simulink model "Ensamblaje_pendulo_furuta_multibody_v4"  (R2025a)
settings: Solver=ode4  StartTime=0.0  StopTime=60  FixedStep=0.002  RelTol=1e-3
PreLoadFcn:
  | d=fileparts(get_param('Ensamblaje_pendulo_furuta_multibody_v4','FileName')); while ~isempty(d)&&~isfile(fullfile(d,'setup_paths.m')), n=fileparts(d); if strcmp(n,d),break;end; d=n; end; if isfile(fullfile(d,'setup_paths.m')), addpath(d); setup_paths; end
  | setup_swingup_quanser; Ensamblaje_pendulo_furuta_multibody_v4_DataFile;
InitFcn:
  | setup_swingup_quanser; Ensamblaje_pendulo_furuta_multibody_v4_DataFile;
model workspace: external: MATLAB File C:\Users\sebas\Documents\TESIS\Scape\Ensamblaje_pendulo_furuta_multibody_v4_DataFile.m (data not in the file)
undefined symbols (not defined in the file): g, Jp_cm, kt, l, mp, mr, r, Rm
libraries: fl_lib x6, simulink_extras x6, nesl_utility x6, simulink x5, sm_lib x2, ee_lib x1
settings Model: Creator=sebas  LastModifiedBy=sebas
settings ExplorerConfigSet: InternalSimMechanicsExplorerSettings=|
  | <ExplorerConfiguration>
  | 
  |   <canonicalview>planar_xy</canonicalview>
  | 
  |   <TilePanel>
  |     <TileInfo>
  |       <Tiles Columns="1" Count="1" Height="592" Rows="1" Width="1064">
  |         <Row Weight="1"/>
  |         <Column Weight="1"/>
  |         <Tile Height="1" Width="1" X="0" Y="0"/>
  |       </Tiles>
  |     </TileInfo>
  |     <SceneInfo>
  |       <SceneViewer>
  |         <IsThisViewStd>
  |           <IsStandardView>off</IsStandardView>
  |           <StandardViewName>Front</StandardViewName>
  |         </IsThisViewStd>
  |         <BGColor>
  |           <R>1</R>
  |           <G>1</G>
  |           <B>1</B>
  |           <A>1</A>
  |         </BGColor>
  |         <Camera>
  |           <DoPerspective>off</DoPerspective>
  |           <Position>
  |             <X>0.15562955258539984</X>
  |             <Y>0.44865320150635074</Y>
  |             <Z>-0.59717677203901176</Z>
  |           </Position>
  |           <Center>
  |             <X>-0.047110070178558651</X>
  |             <Y>0.055245833996093285</Y>
  |             <Z>0.019492845057677309</Z>
  |           </Center>
  |           <Up>
  |             <X>-0.56022370531309607</X>
  |             <Y>0.7694686491141598</Y>
  |             <Z>0.30670408871695148</Z>
  |           </Up>
  |           <XLim>0.11928668495035986</XLim>
  |           <YLim>0.11928668495035986</YLim>
  |           <ViewLimDist>0.01</ViewLimDist>
  |         </Camera>
  |       </SceneViewer>
  |     </SceneInfo>
  |   </TilePanel>
  | 
  |   <MechEditorPanel>
  |     <GfxPanelCameraMap/>
  |     <Cameras/>
  |     <VideoCreator>
  |       <IncludeTiles>All</IncludeTiles>
  |       <IncludeTime>on</IncludeTime>
  |       <IncludeWorldFrame>off</IncludeWorldFrame>
  |       <PlaybackSpeedRatio>1</PlaybackSpeedRatio>
  |       <FrameRate>30</FrameRate>
  |       <FrameSize>auto</FrameSize>
  |       <VideoFormat>UncompressedAVI</VideoFormat>
  |     </VideoCreator>
  |   </MechEditorPanel>
  | 
  |   <PlaybackSettings>
  |     <PlaybackSpeedFactor>1</PlaybackSpeedFactor>
  |   </PlaybackSettings>
  | 
  | </ExplorerConfiguration>

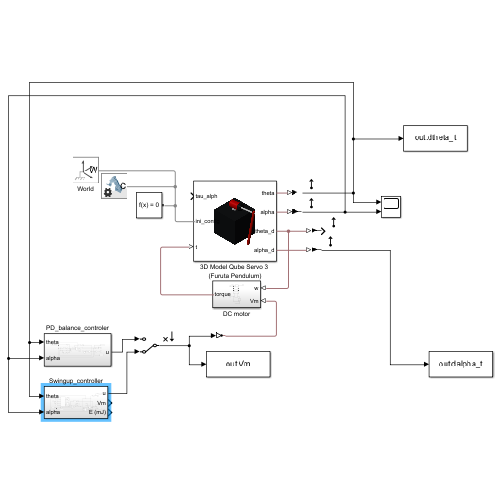
[thumbnail: Simulink's stored preview of the top-level diagram]
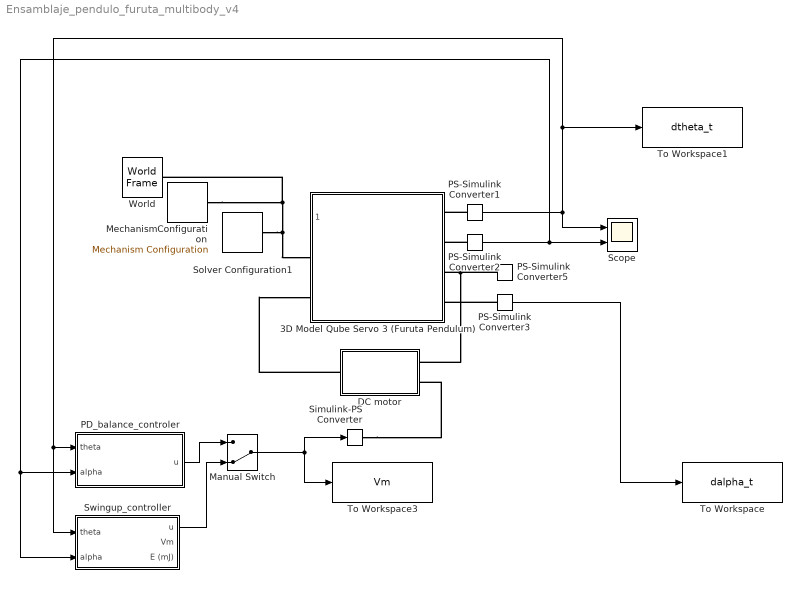
== system Ensamblaje_pendulo_furuta_multibody_v4 ==
  3D Model Qube Servo 3 (Furuta Pendulum) : Subsystem  ReferencedSubsystem=Model3d_Furuta_Pendulum
      settings: PortSchema="{\"entries\":[{\"content\":{\"sides\":[{\"content\":{\"connectorIds\":[\"In1\",\"LConn1\",\"RConn1\"]},\"type\":\"ConnectorPlacement.EquallySpacedRectSide\",\"uuid\":\"a4687828-c9dc-4620-89f9-70fc520029b1\"},{\"content\":{\"connectorIds\":[\"RConn2\",\"RConn3\",\"RConn4\",\"RConn5\"],\"side\":\"RIGHT\"},\"type\":\"ConnectorPlacement.EquallySpacedRectSide\",\"uuid\":\"21a6a3f8-f9ca-4875-ad02-4f645e066fb2\"},{\"content\":{\"side\":\"TOP\"},\"type\":\"ConnectorPlacement.EquallySpacedRectSide\",\"uuid\":\"b064abef-f9ef-4dd8-a3db-595c6ba7d55c\"}]},\"type\":\"ConnectorPlacement.EquallySpacedConnector\",\"uuid\":\"310dfd22-cc79-4c6a-8ca3-9ebbca52c939\"}],\"packageUris\":[\"http://schema.mathworks.com/mf0/Connector/R2020b\"],\"version\":\"1.0\"}"
  DC motor : Subsystem
  Manual Switch : ManualSwitch  CurrentSetting=0
  MechanismConfiguration : sm_lib/Utilities/Mechanism Configuration  UniformGravity=Constant  GravityVector=[0 -9.7807 0]  GravityVectorUnits=m/s^2  LinearizationDelta=0.001  JointModeTransitionNonlinearIterations=2
  PD_balance_controler : Subsystem
  PS-Simulink Converter{1..3,5} (4 alike) : nesl_utility/PS-Simulink Converter  PhysicalDomain=network_engine_domain  SubClassName=ps_output  LeftPortType=input  RightPortType=output  PseudoPeriodic=off  Frequencies=[]  VectorFormat=inherit  Unit=inherit  AffineConversion=off
  Scope : Scope  NumInputPorts=2
      settings: ActiveDisplayYMinimum=-3.5242766671548265  ActiveDisplayYMaximum=3.8832561693672929  DataLoggingVariableName=ScopeData8
  Simulink-PS Converter : nesl_utility/Simulink-PS Converter  PhysicalDomain=network_engine_domain  SubClassName=ps_input  LeftPortType=input  RightPortType=output  PseudoPeriodic=off  Frequencies=[]  NoiseDistribution=none  NoiseParameters=[]  Unit=1  AffineConversion=off  FilteringAndDerivatives=filter  SimscapeFilterOrder=1  InputFilterTimeConstant=0.001  UdotUserProvided=0
  Solver Configuration1 : nesl_utility/Solver Configuration  PhysicalDomain=network_engine_domain  SubClassName=solver  LeftPortType=input  RightPortType=generic  Tones=[]  Harmonics=[]  SimulateNoise=off  Profile=off  UseLocalSampling=off  EnableSwitchedLinearOptims=on  FrequencyDomain=off  UseCCode=off  RelTol=0.001  AbsTol=0.001  MinStep=1e-09  ToWorkspace=off  RevertToSquareIcSolve=off  NumHomotopyIterations=100  PhasorMode=off  PhasorModeNumHarmonics=1  ConsistencySolver=NEWTON_XTOL_AFTER_FTOL  IndexReductionMethod=DerivativeReplacement  DoDC=off  ResidualTolerance=1e-09  ConsistencyTolSource=GLOBAL  ConsistencyAbsTol=0.001  ConsistencyRelTol=0.001  ConsistencyTolFactor=1e-9  UseLocalSolver=on  LocalSolverChoice=NE_BACKWARD_EULER_ADVANCER  ResolveIndetEquations=on  FunctionEvalNumThread=1  LocalSolverSampleTime=0.002  DoFixedCost=on  MaxNonlinIter=5  MaxModeIter=2  ComputeImpulses=on  ImpulseIterations=2  LinearAlgebra=auto  LinearAlgebraNumThread=0  EquationFormulation=NE_TIME_EF  DelaysMemoryBudget=1024  AutomaticFiltering=on  FilteringTimeConstant=0.001  PartitionStorageMethod=AS_NEEDED  PartitionMemoryBudget=1024  PartitionMethod=ROBUST  MultibodyUseLocalSolver=off  MultibodyLocalSolverChoice=ODE1  MultibodyLocalSolverSampleTime=0.002
  Swingup_controller : Subsystem
  To Workspace : ToWorkspace  VariableName=dalpha_t  SampleTime=-1
  To Workspace1 : ToWorkspace  VariableName=dtheta_t  SampleTime=-1
  To Workspace3 : ToWorkspace  VariableName=Vm  SampleTime=-1
  World : sm_lib/Frames and Transforms/World Frame
  wires:
  PD_balance_controler/1(u) -> Manual Switch/1
  Manual Switch/1 -> Simulink-PS Converter/1, To Workspace3/1
  PS-Simulink Converter2/1 -> Swingup_controller/2(alpha), PD_balance_controler/2(alpha), Scope/2
  PS-Simulink Converter1/1 -> To Workspace1/1, Swingup_controller/1(theta), PD_balance_controler/1(theta), Scope/1
  PS-Simulink Converter3/1 -> To Workspace/1
  Swingup_controller/1(u) -> Manual Switch/2
  connections:
  MechanismConfiguration/RConn1 -- Solver Configuration1/RConn1 -- 3D Model Qube Servo 3 (Furuta Pendulum)/LConn1 -- World/RConn1
  PS-Simulink Converter1/LConn1 -- 3D Model Qube Servo 3 (Furuta Pendulum)/RConn2
  PS-Simulink Converter2/LConn1 -- 3D Model Qube Servo 3 (Furuta Pendulum)/RConn3
  DC motor/LConn1 -- 3D Model Qube Servo 3 (Furuta Pendulum)/RConn1
  Simulink-PS Converter/RConn1 -- DC motor/RConn2
  PS-Simulink Converter3/LConn1 -- 3D Model Qube Servo 3 (Furuta Pendulum)/RConn5
  PS-Simulink Converter5/LConn1 -- DC motor/RConn1 -- 3D Model Qube Servo 3 (Furuta Pendulum)/RConn4

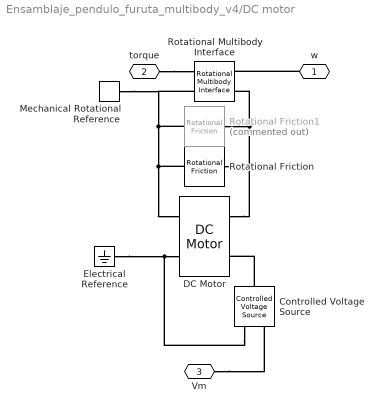
== system Ensamblaje_pendulo_furuta_multibody_v4/DC motor ==
  Controlled Voltage Source : fl_lib/Electrical/Electrical Sources/Controlled Voltage Source
  DC Motor : ee_lib/Electromechanical/Brushed Motors/DC Motor  field_option=ee.enum.field_option.pm  Rf=100 Ohm  Lf=1 H  Laf=0.15 H  If0=0 A  parameterization=ee.enum.dcparam_option.circuit_param  Ra=7.5 Ohm  La=1.15e-3 H  emf_or_torque=ee.enum.emf_or_torque.kv  Kv=0.0422 V*s/rad  Ki=0.0422 N*m/A  T_stall=0.24e-3 N*m  w_max=5400 rpm  w_rated=4579 rpm  P_rated=9.8 W  V_rated=24 V  lam_param=ee.enum.lam_param.damping  i_noload=16 mA  V_i_noload=24 V  J=1.4e-6 kg*m^2  lam=1*4.8390e-6 N*m*s/rad  speed0=0 rpm  alpha=3.93e-3 1/K  Tmeas=25 degC  thermal_mass=100 J/K  initial_temperature=25 degC
  Electrical Reference : fl_lib/Electrical/Electrical Elements/Electrical Reference
  Mechanical Rotational Reference : fl_lib/Mechanical/Rotational Elements/Mechanical Rotational Reference
  Rotational Friction : fl_lib/Mechanical/Rotational Elements/Rotational Friction  brkwy_trq=1*2.910555e-05+1*4.081637e-05 N*m  brkwy_vel=1.082312e-02 rad/s  Col_trq=2.910555e-05 N*m  visc_coef=4.321929e-06 N*m*s/rad  w_specify=off  w_priority=None  w=0 rad/s  w_nominal_specify=off  w_nominal_value=1  w_nominal_unit=rad/s  t_specify=off  t_priority=None  t=0 N*m  t_nominal_specify=off  t_nominal_value=1  t_nominal_unit=N*m
  Rotational Friction1 : fl_lib/Mechanical/Rotational Elements/Rotational Friction  Commented=on  brkwy_trq=7.066e-04 N*m  brkwy_vel=0.1 rad/s  Col_trq=7.066e-09 N*m  visc_coef=0 N*m*s/rad  w_specify=off  w_priority=None  w=0 rad/s  w_nominal_specify=off  w_nominal_value=1  w_nominal_unit=rad/s  t_specify=off  t_priority=None  t=0 N*m  t_nominal_specify=off  t_nominal_value=1  t_nominal_unit=N*m
  Rotational Multibody Interface : fl_lib/Mechanical/Multibody Interfaces/Rotational Multibody Interface
  w : PMIOPort  Side=Right
  torque : PMIOPort  Port=2  Side=Left
  Vm : PMIOPort  Port=3  Side=Right
  connections:
  Rotational Friction/LConn1 -- DC Motor/LConn2 -- Rotational Friction1/LConn1 -- Rotational Multibody Interface/RConn2
  torque/RConn1 -- Rotational Multibody Interface/LConn1
  Rotational Friction/RConn1 -- Rotational Friction1/RConn1 -- Rotational Multibody Interface/LConn2 -- Mechanical Rotational Reference/LConn1 -- DC Motor/RConn2
  Vm/RConn1 -- Controlled Voltage Source/RConn1
  w/RConn1 -- Rotational Multibody Interface/RConn1
  DC Motor/RConn1 -- Electrical Reference/LConn1 -- Controlled Voltage Source/RConn2
  Controlled Voltage Source/LConn1 -- DC Motor/LConn1

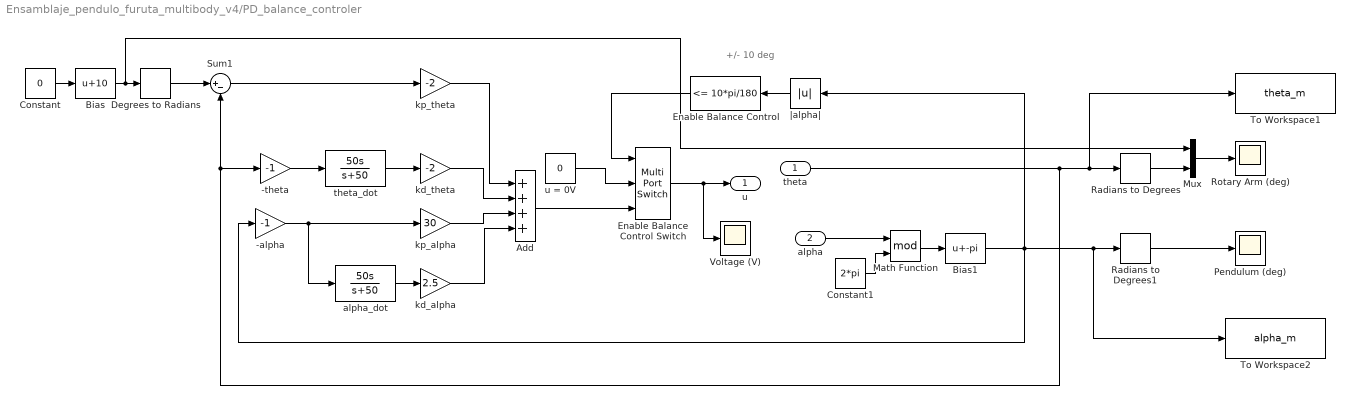
== system Ensamblaje_pendulo_furuta_multibody_v4/PD_balance_controler ==
  note: +/- 10 deg
  theta : Inport
  alpha : Inport  Port=2
  -alpha : Gain  Gain=-1
  -theta : Gain  Gain=-1
  Add : Sum  Inputs=++++
  Bias : Bias  Bias=10  SaturateOnIntegerOverflow=off
  Bias1 : Bias  Bias=-pi  SaturateOnIntegerOverflow=off
  Constant : Constant  Value=0
  Constant1 : Constant  Value=2*pi
  Degrees to Radians : simulink_extras/Transformations/Degrees to Radians
  Enable Balance Control : simulink/Logic and Bit Operations/Compare To Constant  relop=<=  const=10*pi/180  OutDataTypeStr=uint8  ZeroCross=off
  Enable Balance Control Switch : MultiPortSwitch  DataPortOrder=Zero-based contiguous  Inputs=2  zeroidx=on  SaturateOnIntegerOverflow=off  InputSameDT=off
  Math Function : Math  Operator=mod  SignedPower=on
  Mux : Mux  Inputs=2
  Pendulum (deg) : Scope
      settings: ActiveDisplayYMinimum=-1.7148524393471249  ActiveDisplayYMaximum=1.4022626573328889
  Radians to Degrees : simulink_extras/Transformations/Radians to Degrees
  Radians to Degrees1 : simulink_extras/Transformations/Radians to Degrees
  Rotary Arm (deg) : Scope
      settings: ActiveDisplayYMinimum=-20.263400075625345  ActiveDisplayYMaximum=153.53436969880661
  Sum1 : Sum  Inputs=|+-
  To Workspace1 : ToWorkspace  VariableName=theta_m  SampleTime=-1
  To Workspace2 : ToWorkspace  VariableName=alpha_m  SampleTime=-1
  Voltage (V) : Scope
      settings: ActiveDisplayYMinimum=-1  ActiveDisplayYMaximum=1  DataLoggingVariableName=ScopeData2
  alpha_dot : TransferFcn  Numerator=[50 0]  Denominator=[1 50]
  kd_alpha : Gain  Gain=2.5
  kd_theta : Gain  Gain=-2
  kp_alpha : Gain  Gain=30
  kp_theta : Gain  Gain=-2
  theta_dot : TransferFcn  Numerator=[50 0]  Denominator=[1 50]
  u = 0V : Constant  Value=0
  |alpha| : Abs  SaturateOnIntegerOverflow=off
  u : Outport
  wires:
  alpha/1 -> Math Function/1
  Constant1/1 -> Math Function/2
  Math Function/1 -> Bias1/1
  Bias1/1 -> To Workspace2/1, Radians to Degrees1/1, |alpha|/1, -alpha/1
  Constant/1 -> Bias/1
  Add/1 -> Enable Balance Control Switch/3
  -theta/1 -> theta_dot/1
  |alpha|/1 -> Enable Balance Control/1
  Radians to Degrees1/1 -> Pendulum (deg)/1
  kp_theta/1 -> Add/1
  alpha_dot/1 -> kd_alpha/1
  Radians to Degrees/1 -> Mux/2
  kd_theta/1 -> Add/2
  theta/1 -> To Workspace1/1, Radians to Degrees/1, Sum1/2, -theta/1
  theta_dot/1 -> kd_theta/1
  Bias/1 -> Degrees to Radians/1, Mux/1
  Degrees to Radians/1 -> Sum1/1
  u = 0V/1 -> Enable Balance Control Switch/2
  -alpha/1 -> alpha_dot/1, kp_alpha/1
  Mux/1 -> Rotary Arm (deg)/1
  kp_alpha/1 -> Add/3
  Sum1/1 -> kp_theta/1
  Enable Balance Control/1 -> Enable Balance Control Switch/1
  kd_alpha/1 -> Add/4
  Enable Balance Control Switch/1 -> u/1, Voltage (V)/1

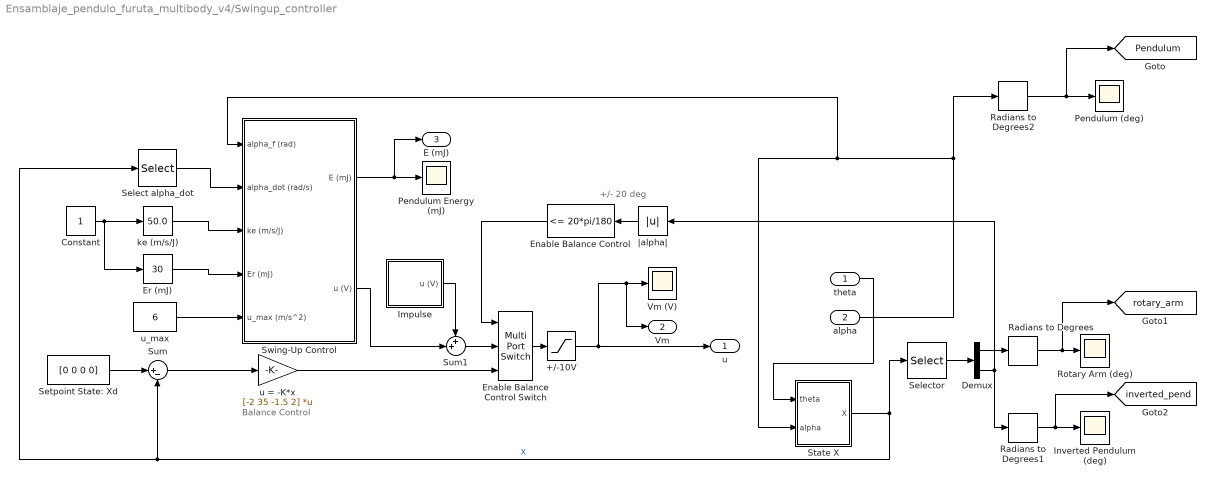
== system Ensamblaje_pendulo_furuta_multibody_v4/Swingup_controller ==
  note: Balance Control
  note: +/- 20 deg
  theta : Inport
  alpha : Inport  Port=2
  +/-10V : Saturate  UpperLimit=10  LowerLimit=-10
  Constant : Constant
  Demux : Demux  Outputs=2
  Enable Balance Control : simulink/Logic and Bit Operations/Compare To Constant  relop=<=  const=20*pi/180  OutDataTypeStr=uint8  ZeroCross=off
  Enable Balance Control Switch : MultiPortSwitch  DataPortOrder=Zero-based contiguous  Inputs=2  zeroidx=on  SaturateOnIntegerOverflow=off  InputSameDT=off
  Er (mJ) : simulink/Math Operations/Slider Gain  gain=30  low=0  high=100
  Impulse : Subsystem
  Inverted Pendulum (deg) : Scope
      settings: ActiveDisplayYMinimum=-224.99984832258403  ActiveDisplayYMaximum=224.99863490325629  DataLoggingVariableName=ScopeData4
  Pendulum (deg) : Scope
      settings: ActiveDisplayYMinimum=-200.66195430718761  ActiveDisplayYMaximum=222.65973832089497  DataLoggingVariableName=ScopeData5  DataLoggingSaveFormat=Array
  Pendulum Energy (mJ) : Scope
      settings: ActiveDisplayYMinimum=-1.7076335355968837  ActiveDisplayYMaximum=4.1343640569805871  DataLoggingVariableName=ScopeData3
  Radians to Degrees : simulink_extras/Transformations/Radians to Degrees
  Radians to Degrees1 : simulink_extras/Transformations/Radians to Degrees
  Radians to Degrees2 : simulink_extras/Transformations/Radians to Degrees
  Rotary Arm (deg) : Scope
      settings: ActiveDisplayYMinimum=-50.204630202298013  ActiveDisplayYMaximum=96.919601983870734  DataLoggingVariableName=ScopeData6
  Select alpha_dot : Selector  InputPortWidth=4  IndexOptions=Index vector (dialog)  Indices=[4]  OutputSizes=1
  Selector : Selector  InputPortWidth=4  IndexOptions=Index vector (dialog)  Indices=[1 2]  OutputSizes=1
  Setpoint State: Xd : Constant  Value=[0 0 0 0]
  State X : Subsystem
  Sum : Sum  Inputs=|+-
  Sum1 : Sum  Inputs=++|
  Swing-Up Control : Subsystem
  Vm (V) : Scope
      settings: ActiveDisplayYMinimum=-6.7281905852078392  ActiveDisplayYMaximum=10.042270651945255  DataLoggingVariableName=ScopeData7
  ke (m/s/J) : simulink/Math Operations/Slider Gain  gain=50.0  low=0  high=100
  u = -K*x : Gain  Gain=[-2 35 -1.5 2]  Multiplication=Matrix(K*u)
  u_max : Constant  Value=6
  |alpha| : Abs  SaturateOnIntegerOverflow=off
  u : Outport
  Vm : Outport  Port=2
  E (mJ) : Outport  Port=3
  tag scope: Pendulum=global, inverted_pend=global, rotary_arm=global
  wires:
  alpha/1 -> State X/2(alpha), Swing-Up Control/1(alpha_f (rad)), Radians to Degrees2/1
  Sum1/1 -> Enable Balance Control Switch/2
  Selector/1 -> Demux/1
  Enable Balance Control/1 -> Enable Balance Control Switch/1
  Sum/1 -> u = -K*x/1
  u_max/1 -> Swing-Up Control/5(u_max (m/s^2))
  |alpha|/1 -> Enable Balance Control/1
  Impulse/1(u (V)) -> Sum1/1
  Swing-Up Control/1(E (mJ)) -> E (mJ)/1, Pendulum Energy (mJ)/1
  u = -K*x/1 -> Enable Balance Control Switch/3
  Radians to Degrees/1 -> [rotary_arm], Rotary Arm (deg)/1
  Demux/2 -> Radians to Degrees1/1, |alpha|/1
  Swing-Up Control/2(u (V)) -> Sum1/2
  Radians to Degrees2/1 -> [Pendulum], Pendulum (deg)/1
  ke (m/s/J)/1 -> Swing-Up Control/3(ke (m/s/J))
  Enable Balance Control Switch/1 -> +/-10V/1
  +/-10V/1 -> u/1, Vm/1, Vm (V)/1
  theta/1 -> State X/1(theta)
  Radians to Degrees1/1 -> [inverted_pend], Inverted Pendulum (deg)/1
  Constant/1 -> Er (mJ)/1, ke (m/s/J)/1
  State X/1(X) -> Sum/2, Select alpha_dot/1, Selector/1  "X"
  Setpoint State: Xd/1 -> Sum/1
  Demux/1 -> Radians to Degrees/1
  Er (mJ)/1 -> Swing-Up Control/4(Er (mJ))
  Select alpha_dot/1 -> Swing-Up Control/2(alpha_dot (rad/s))

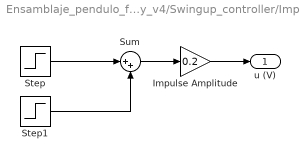
== system Ensamblaje_pendulo_furuta_multibody_v4/Swingup_controller/Impulse ==
  Impulse Amplitude : Gain  Gain=0.2
  Step : Step  SampleTime=0
  Step1 : Step  Time=1.1  After=-1  SampleTime=0
  Sum : Sum  Inputs=|++
  u (V) : Outport  VectorParamsAs1DForOutWhenUnconnected=off
  wires:
  Impulse Amplitude/1 -> u (V)/1
  Sum/1 -> Impulse Amplitude/1
  Step/1 -> Sum/1
  Step1/1 -> Sum/2

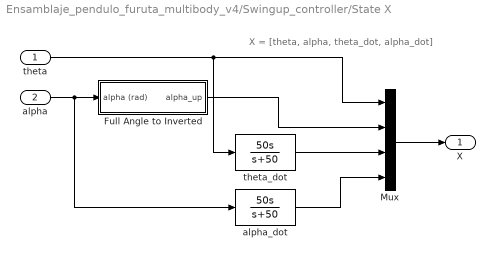
== system Ensamblaje_pendulo_furuta_multibody_v4/Swingup_controller/State X ==
  note: X = [theta, alpha, theta_dot, alpha_dot]
  theta : Inport
  alpha : Inport  Port=2
  Full Angle to Inverted : Subsystem
  Mux : Mux
  alpha_dot : TransferFcn  Numerator=[50 0]  Denominator=[1 50]
  theta_dot : TransferFcn  Numerator=[50 0]  Denominator=[1 50]
  X : Outport  VectorParamsAs1DForOutWhenUnconnected=off
  wires:
  Full Angle to Inverted/1(alpha_up) -> Mux/2
  alpha_dot/1 -> Mux/4
  theta_dot/1 -> Mux/3
  theta/1 -> Mux/1, theta_dot/1
  alpha/1 -> alpha_dot/1, Full Angle to Inverted/1(alpha (rad))
  Mux/1 -> X/1

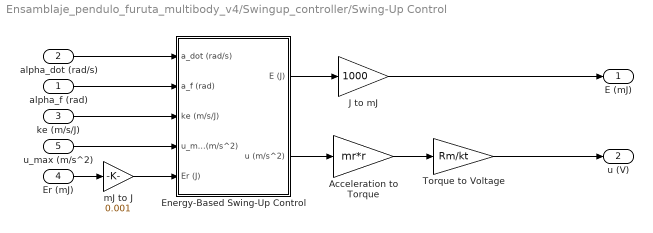
== system Ensamblaje_pendulo_furuta_multibody_v4/Swingup_controller/Swing-Up Control ==
  alpha_f (rad) : Inport
  alpha_dot (rad/s) : Inport  Port=2
  ke (m/s/J) : Inport  Port=3
  Er (mJ) : Inport  Port=4
  u_max (m/s^2) : Inport  Port=5
  Acceleration to Torque : Gain  Gain=mr*r
  Energy-Based Swing-Up Control : Subsystem
  J to mJ : Gain  Gain=1000
  Torque to Voltage : Gain  Gain=Rm/kt
  mJ to J : Gain  Gain=0.001
  E (mJ) : Outport  VectorParamsAs1DForOutWhenUnconnected=off
  u (V) : Outport  Port=2  VectorParamsAs1DForOutWhenUnconnected=off
  wires:
  mJ to J/1 -> Energy-Based Swing-Up Control/5(Er (J))
  alpha_dot (rad/s)/1 -> Energy-Based Swing-Up Control/1(a_dot (rad/s))
  Torque to Voltage/1 -> u (V)/1
  J to mJ/1 -> E (mJ)/1
  Er (mJ)/1 -> mJ to J/1
  Acceleration to Torque/1 -> Torque to Voltage/1
  u_max (m/s^2)/1 -> Energy-Based Swing-Up Control/4(u_max (m/s^2))
  ke (m/s/J)/1 -> Energy-Based Swing-Up Control/3(ke (m/s/J))
  alpha_f (rad)/1 -> Energy-Based Swing-Up Control/2(a_f (rad))
  Energy-Based Swing-Up Control/1(E (J)) -> J to mJ/1
  Energy-Based Swing-Up Control/2(u (m/s^2)) -> Acceleration to Torque/1

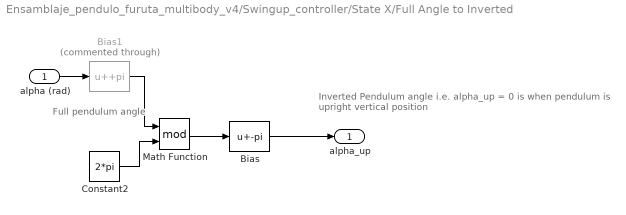
== system Ensamblaje_pendulo_furuta_multibody_v4/Swingup_controller/State X/Full Angle to Inverted ==
  note: Full pendulum angle
  note: Inverted Pendulum angle
      | i.e. alpha_up = 0 is when pendulum is upright vertical position
  alpha (rad) : Inport
  Bias : Bias  Bias=-pi  SaturateOnIntegerOverflow=off
  Bias1 : Bias  Commented=through  Bias=+pi  SaturateOnIntegerOverflow=off
  Constant2 : Constant  Value=2*pi
  Math Function : Math  Operator=mod  SignedPower=on
  alpha_up : Outport  VectorParamsAs1DForOutWhenUnconnected=off
  wires:
  Bias1/1 -> Math Function/1
  Math Function/1 -> Bias/1
  Bias/1 -> alpha_up/1
  alpha (rad)/1 -> Bias1/1
  Constant2/1 -> Math Function/2

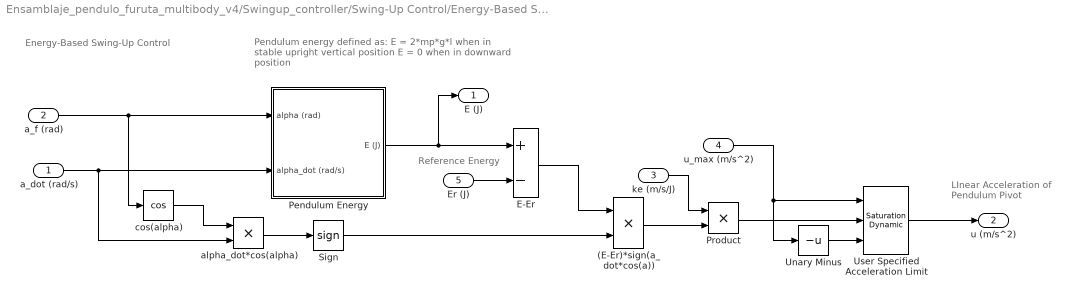
== system Ensamblaje_pendulo_furuta_multibody_v4/Swingup_controller/Swing-Up Control/Energy-Based Swing-Up Control ==
  note: Pendulum energy defined as:
      | E = 2*mp*g*l when in stable upright vertical position
      | E = 0 when in downward position
  note: Reference Energy
  note: LInear Acceleration of
      | Pendulum Pivot
  note: Energy-Based Swing-Up Control
  a_dot (rad/s) : Inport
  a_f (rad) : Inport  Port=2
  ke (m/s/J) : Inport  Port=3
  u_max (m/s^2) : Inport  Port=4
  Er (J) : Inport  Port=5
  (E-Er)*sign(a_dot*cos(a)) : Product  RndMeth=Zero
  E-Er : Sum  Inputs=+-
  Pendulum Energy : Subsystem
  Product : Product  RndMeth=Zero
  Sign : Signum
  Unary Minus : UnaryMinus
  User Specified Acceleration Limit : simulink/Discontinuities/Saturation Dynamic  OutMin=[]  OutMax=[]  OutDataTypeStr=Inherit: Same as second input  OutDataType=fixdt(1, 16)  OutScaling=2^-10  DoSatur=off
  alpha_dot*cos(alpha) : Product  RndMeth=Zero
  cos(alpha) : Trigonometry  Operator=cos
  E (J) : Outport  VectorParamsAs1DForOutWhenUnconnected=off
  u (m/s^2) : Outport  Port=2  VectorParamsAs1DForOutWhenUnconnected=off
  wires:
  User Specified Acceleration Limit/1 -> u (m/s^2)/1
  Unary Minus/1 -> User Specified Acceleration Limit/3
  u_max (m/s^2)/1 -> Unary Minus/1, User Specified Acceleration Limit/1
  Product/1 -> User Specified Acceleration Limit/2
  ke (m/s/J)/1 -> Product/1
  Er (J)/1 -> E-Er/2
  (E-Er)*sign(a_dot*cos(a))/1 -> Product/2
  a_dot (rad/s)/1 -> Pendulum Energy/2(alpha_dot (rad/s)), alpha_dot*cos(alpha)/2
  Pendulum Energy/1(E (J)) -> E-Er/1, E (J)/1
  E-Er/1 -> (E-Er)*sign(a_dot*cos(a))/1
  cos(alpha)/1 -> alpha_dot*cos(alpha)/1
  alpha_dot*cos(alpha)/1 -> Sign/1
  Sign/1 -> (E-Er)*sign(a_dot*cos(a))/2
  a_f (rad)/1 -> cos(alpha)/1, Pendulum Energy/1(alpha (rad))

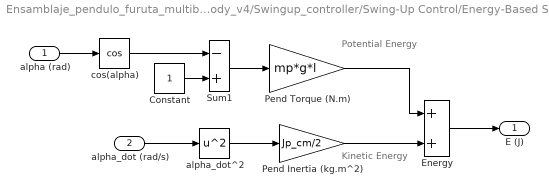
== system Ensamblaje_pendulo_furuta_multibody_v4/Swingup_controller/Swing-Up Control/Energy-Based Swing-Up Control/Pendulum Energy ==
  note: Potential Energy
  note: Kinetic Energy
  alpha (rad) : Inport
  alpha_dot (rad/s) : Inport  Port=2
  Constant : Constant
  Energy : Sum  SaturateOnIntegerOverflow=on
  Pend Inertia (kg.m^2) : Gain  Gain=Jp_cm/2
  Pend Torque (N.m) : Gain  Gain=mp*g*l
  Sum1 : Sum  Inputs=-+  SaturateOnIntegerOverflow=on
  alpha_dot^2 : Math  Operator=square  SignedPower=on
  cos(alpha) : Trigonometry  Operator=cos
  E (J) : Outport  VectorParamsAs1DForOutWhenUnconnected=off
  wires:
  cos(alpha)/1 -> Sum1/1
  Energy/1 -> E (J)/1
  alpha_dot (rad/s)/1 -> alpha_dot^2/1
  alpha (rad)/1 -> cos(alpha)/1
  Pend Torque (N.m)/1 -> Energy/1
  alpha_dot^2/1 -> Pend Inertia (kg.m^2)/1
  Pend Inertia (kg.m^2)/1 -> Energy/2
  Constant/1 -> Sum1/2
  Sum1/1 -> Pend Torque (N.m)/1
